simulink model "FUZZY_T2_ADRC_P3DX"  (R2024b)
settings: Solver=FixedStepAuto  StartTime=0.0  StopTime=16  FixedStep=0.01  RelTol=1e-2
libraries: fuzblock x2, simulink x1
settings Model: Creator=Dell  LastModifiedBy=Dell
settings DebuggingCC: AlgebraicLoopMsg=none  SigSpecEnsureSampleTimeMsg=none
settings RTWCC: GPUComputeCapability=3.5

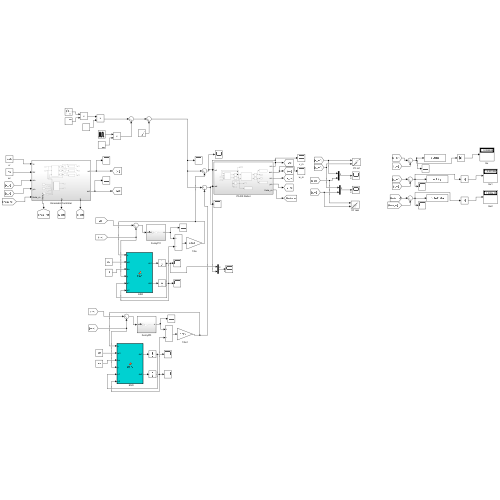
[thumbnail: Simulink's stored preview of the top-level diagram]
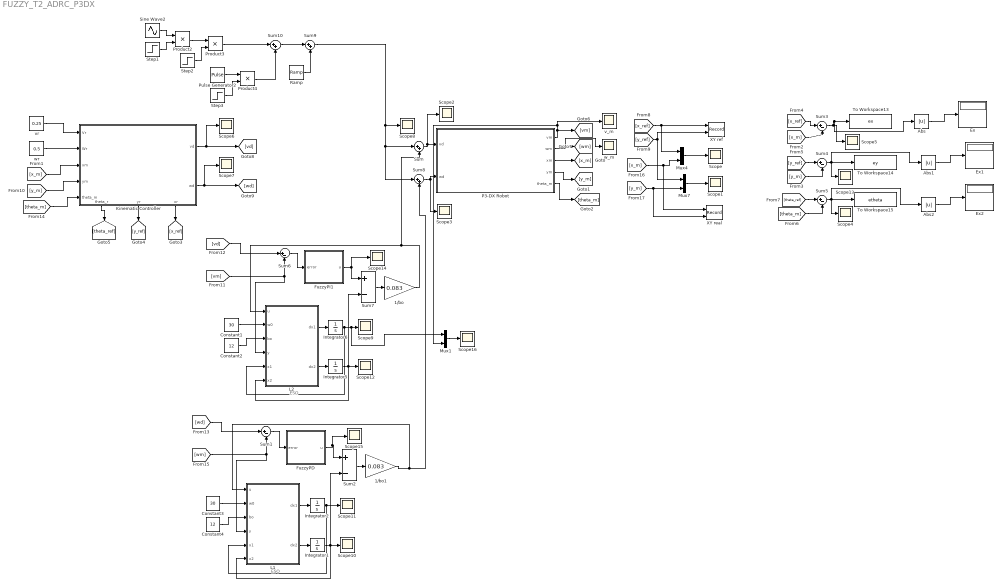
== system FUZZY_T2_ADRC_P3DX ==
  note: ESO
  note: ESO
  1/bo : Gain  Gain=0.083
  1/bo1 : Gain  Gain=0.083
  Abs : Abs  SaturateOnIntegerOverflow=off
  Abs1 : Abs  SaturateOnIntegerOverflow=off
  Abs2 : Abs  SaturateOnIntegerOverflow=off
  Constant1 : Constant  Value=30
  Constant2 : Constant  Value=12
  Constant3 : Constant  Value=30
  Constant4 : Constant  Value=12
  Ex : Display
  Ex1 : Display
  Ex2 : Display
  FuzzyPD : Subsystem
  FuzzyPI1 : Subsystem
  Integrator{1..2,5..6} (4 alike) : Integrator
  Kinematic Controller : Subsystem
      settings: PortSchema="{\"entries\":[{\"content\":{\"sides\":[{\"content\":{\"connectorIds\":[\"In1\",\"In2\",\"In3\",\"In4\",\"In5\"]},\"type\":\"ConnectorPlacement.EquallySpacedRectSide\",\"uuid\":\"1dde3c4d-b362-4c98-bff5-173134d67a18\"},{\"content\":{\"connectorIds\":[\"Out1\",\"Out2\"],\"side\":\"RIGHT\"},\"type\":\"ConnectorPlacement.EquallySpacedRectSide\",\"uuid\":\"28a7b07a-1542-4ec6-930a-70e18e33702f\"},{\"content\":{\"side\":\"TOP\"},\"type\":\"ConnectorPlacement.EquallySpacedRectSide\",\"uuid\":\"fddfb50e-6b1f-4e7e-bd72-f809cd3d8285\"},{\"content\":{\"connectorIds\":[\"Out3\",\"Out4\",\"Out5\"],\"side\":\"BOTTOM\"},\"type\":\"ConnectorPlacement.EquallySpacedRectSide\",\"uuid\":\"0cbc9f95-9386-4a92-999a-6cc6855b0431\"}]},\"type\":\"ConnectorPlacement.EquallySpacedConnector\",\"uuid\":\"21383b85-61ab-4832-be46-2fedf08e757e\"}],\"packageUris\":[\"http://schema.mathworks.com/mf0/Connector/R2020b\"],\"version\":\"1.0\"}"
  L1 : MATLAB Function  TreatAsAtomicUnit=on
  L2 : MATLAB Function  TreatAsAtomicUnit=on
  Mux1 : Mux  Inputs=2
  Mux4 : Mux  Inputs=2
  Mux7 : Mux  Inputs=2
  P3-DX Robot : Subsystem
  Product2 : Product
  Product3 : Product
  Product4 : Product
  Pulse Generator2 : DiscretePulseGenerator  PulseType=Time based  Amplitude=4  Period=1  PulseWidth=35  PhaseDelay=9.7
  Ramp : simulink/Sources/Ramp  slope=1  start=14.3  InitialOutput=0
  Scope{,1..16} (17 alike) : Scope
  Sine Wave2 : Sin  Amplitude=4  Frequency=2  SampleTime=0
  Step1 : Step  Time=3.2  SampleTime=0
  Step2 : Step  Time=9.4  Before=1  After=0  SampleTime=0
  Step3 : Step  Time=14  Before=1  After=0  SampleTime=0
  Sum{,8..10} (4 alike) : Sum  Inputs=|++
  Sum{1,3..6} (5 alike) : Sum  Inputs=|+-
  Sum2 : Sum  Inputs=+-
  Sum7 : Sum  Inputs=+-
  To Workspace13 : ToWorkspace  VariableName=ex  SaveFormat=Timeseries  SampleTime=-1
  To Workspace14 : ToWorkspace  VariableName=ey  SaveFormat=Timeseries  SampleTime=-1
  To Workspace15 : ToWorkspace  VariableName=etheta  SaveFormat=Timeseries  SampleTime=-1
  XY real : Record  FileSettingsInternal="{\"entries\":[{\"content\":{\"excelSettings\":{\"content\":{},\"type\":\"Streamout.ExcelSettings\"}},\"type\":\"Streamout.FileSettingStorage\",\"uuid\":\"\"}],\"packageUris\":[\"http:\\/\\/schema.mathworks.com\\/mf0\\/streamout_blocks\\/R2020a\"],\"version\":\"1.0\"}"  Layout=[1 1]  SignalsInternal="{\"entries\":[{\"content\":{\"signals\":[{\"content\":{\"blockPath\":[],\"dimensions\":[1],\"domain\":\"\",\"lineColor\":\"#139fff\",\"lineWidth\":2,\"port\":1,\"sid\":[\"\"],\"signalID\":1,\"signalName\":\"From16\"},\"type\":\"RecordBlkView.Signal\",\"uuid\":\"\"},{\"content\":{\"blockPath\":[],\"dimensions\":[1],\"domain\":\"\",\"lineColor\":\"#ff6929\",\"lineWidth\":2,\"port\":2,\"sid\":[\"\"],\"signalID\":2,\"signalName\":\"From17\"},\"type\":\"RecordBlkView.Signal\",\"uuid\":\"\"}]},\"type\":\"RecordBlkView.InputSignals\",\"uuid\":\"\"}],\"packageUris\":[\"http:\\/\\/schema.mathworks.com\\/mf0\\/streamout_blocks\\/R2020a\"],\"version\":\"1.0\"}"  VisualizationBindings="{\"xyplotplugin\":{\"info\":[{\"series\":[],\"subplotID\":1}]}}"  CompatibilityTag=XY
  XY ref : Record  FileSettingsInternal="{\"entries\":[{\"content\":{\"excelSettings\":{\"content\":{},\"type\":\"Streamout.ExcelSettings\"}},\"type\":\"Streamout.FileSettingStorage\",\"uuid\":\"\"}],\"packageUris\":[\"http:\\/\\/schema.mathworks.com\\/mf0\\/streamout_blocks\\/R2020a\"],\"version\":\"1.0\"}"  Layout=[1 1]  SignalsInternal="{\"entries\":[{\"content\":{\"signals\":[{\"content\":{\"blockPath\":[],\"dimensions\":[1],\"domain\":\"\",\"lineColor\":\"#b746ff\",\"lineWidth\":2,\"port\":1,\"sid\":[\"\"],\"signalID\":1,\"signalName\":\"From8\"},\"type\":\"RecordBlkView.Signal\",\"uuid\":\"\"},{\"content\":{\"blockPath\":[],\"dimensions\":[1],\"domain\":\"\",\"lineColor\":\"#64d413\",\"lineWidth\":2,\"port\":2,\"sid\":[\"\"],\"signalID\":2,\"signalName\":\"From9\"},\"type\":\"RecordBlkView.Signal\",\"uuid\":\"\"}]},\"type\":\"RecordBlkView.InputSignals\",\"uuid\":\"\"}],\"packageUris\":[\"http:\\/\\/schema.mathworks.com\\/mf0\\/streamout_blocks\\/R2020a\"],\"version\":\"1.0\"}"  VisualizationBindings="{\"xyplotplugin\":{\"info\":[{\"series\":[],\"subplotID\":1}]}}"  CompatibilityTag=XY
  v_m : Scope
  vr : Constant  Value=0.25
  w_m : Scope
  wr : Constant  Value=0.5
  wires:
  Abs1/1 -> Ex1/1
  Abs/1 -> Ex/1
  [y_ref] -> Sum4/1
  [x_m] -> Sum3/2
  [theta_m] -> Sum5/2
  Sum5/1 -> Abs2/1, Scope4/1, To Workspace15/1
  Sum3/1 -> Abs/1, To Workspace13/1, Scope5/1
  [theta_ref] -> Sum5/1
  Abs2/1 -> Ex2/1
  [y_m] -> Sum4/2
  [x_ref] -> Sum3/1
  Sum4/1 -> Abs1/1, Scope13/1, To Workspace14/1
  Mux4/1 -> Scope/1
  Mux7/1 -> Scope1/1
  [y_ref] -> XY ref/2, Mux7/1
  [x_ref] -> XY ref/1, Mux4/1
  [x_m] -> XY real/1, Mux4/2
  [y_m] -> XY real/2, Mux7/2
  [y_m] -> Kinematic Controller/4(ym)
  vr/1 -> Kinematic Controller/1(Vr)
  wr/1 -> Kinematic Controller/2(Wr)
  [x_m] -> Kinematic Controller/3(xm)
  [theta_m] -> Kinematic Controller/5(theta_m)
  P3-DX Robot/3(xm) -> [x_m]
  P3-DX Robot/4(ym) -> [y_m]
  P3-DX Robot/5(theta_m) -> [theta_m]
  Kinematic Controller/5(xr) -> [x_ref]
  Kinematic Controller/4(yr) -> [y_ref]
  Kinematic Controller/3(theta_r) -> [theta_ref]
  P3-DX Robot/1(vm) -> Mux1/2, v_m/1, [vm]
  Kinematic Controller/2(wd) -> [wd], Scope7/1
  P3-DX Robot/2(wm) -> w_m/1, [wm]
  Kinematic Controller/1(vd) -> [vd], Scope6/1
  1/bo/1 -> Sum/2, L2/1(u)
  Constant2/1 -> L2/3(bo)
  [vd] -> Sum6/1
  Integrator6/1 -> L2/5(x1), Mux1/1, Scope9/1
  Sum7/1 -> 1/bo/1
  [vm] -> L2/4(y), Sum6/2
  Constant1/1 -> L2/2(w0)
  Integrator5/1 -> Sum7/2, Scope12/1, L2/6(x2)
  L2/2(dx2) -> Integrator5/1
  L2/1(dx1) -> Integrator6/1
  L1/2(dx2) -> Integrator1/1
  Integrator1/1 -> Sum2/2, Scope10/1, L1/6(x2)
  [wm] -> L1/4(y), Sum1/2
  Constant3/1 -> L1/2(w0)
  Sum2/1 -> 1/bo1/1
  Integrator2/1 -> L1/5(x1), Scope11/1
  L1/1(dx1) -> Integrator2/1
  [wd] -> Sum1/1
  Constant4/1 -> L1/3(bo)
  1/bo1/1 -> Sum8/2, L1/1(u)
  Sum/1 -> Scope2/1, P3-DX Robot/1(vd)
  Sum8/1 -> Scope3/1, P3-DX Robot/2(wd)
  Sum1/1 -> FuzzyPD/1(error)
  FuzzyPD/1(u) -> Scope15/1, Sum2/1
  Sum9/1 -> Sum8/1, Sum/1, Scope8/1
  Pulse Generator2/1 -> Product4/1
  Ramp/1 -> Sum9/2
  Sine Wave2/1 -> Product2/1
  Step1/1 -> Product2/2
  Step2/1 -> Product3/2
  Product4/1 -> Sum10/2
  Sum10/1 -> Sum9/1
  Step3/1 -> Product4/2
  Product3/1 -> Sum10/1
  Product2/1 -> Product3/1
  Sum6/1 -> FuzzyPI1/1(error)
  FuzzyPI1/1(u) -> Sum7/1, Scope14/1
  Mux1/1 -> Scope16/1

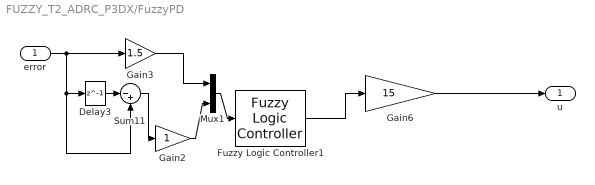
== system FUZZY_T2_ADRC_P3DX/FuzzyPD ==
  error : Inport
  Delay3 : Delay  DelayLength=1  InitialCondition=0
  Fuzzy Logic Controller1 : fuzblock/Fuzzy Logic  Controller  FIS='PI_type2.fis'  OutputSampleNumber=101  DataType=double  FuzzifiedInputs=off  RuleFiringStrengths=off  RuleOutputs=off  AggregatedOutputs=off  SimulateUsing=Interpreted execution  OutOfRangeInputValueMessage=warning  NoRuleFiredMessage=warning  EmptyOutputFuzzySetMessage=warning
  Gain2 : Gain
  Gain3 : Gain  Gain=1.5
  Gain6 : Gain  Gain=15
  Mux1 : Mux  Inputs=2
  Sum11 : Sum  Inputs=|-+
  u : Outport
  wires:
  error/1 -> Gain3/1, Sum11/2, Delay3/1
  Delay3/1 -> Sum11/1
  Sum11/1 -> Gain2/1
  Gain2/1 -> Mux1/2
  Mux1/1 -> Fuzzy Logic Controller1/1
  Fuzzy Logic Controller1/1 -> Gain6/1
  Gain3/1 -> Mux1/1
  Gain6/1 -> u/1

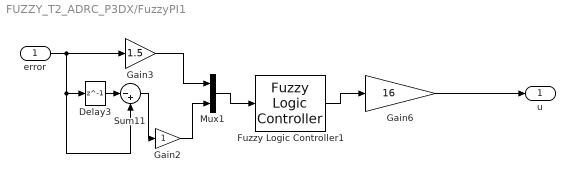
== system FUZZY_T2_ADRC_P3DX/FuzzyPI1 ==
  error : Inport
  Delay3 : Delay  DelayLength=1  InitialCondition=0
  Fuzzy Logic Controller1 : fuzblock/Fuzzy Logic  Controller  FIS='PI_type2.fis'  OutputSampleNumber=101  DataType=double  FuzzifiedInputs=off  RuleFiringStrengths=off  RuleOutputs=off  AggregatedOutputs=off  SimulateUsing=Interpreted execution  OutOfRangeInputValueMessage=warning  NoRuleFiredMessage=warning  EmptyOutputFuzzySetMessage=warning
  Gain2 : Gain
  Gain3 : Gain  Gain=1.5
  Gain6 : Gain  Gain=16
  Mux1 : Mux  Inputs=2
  Sum11 : Sum  Inputs=|-+
  u : Outport
  wires:
  error/1 -> Gain3/1, Sum11/2, Delay3/1
  Delay3/1 -> Sum11/1
  Sum11/1 -> Gain2/1
  Gain2/1 -> Mux1/2
  Mux1/1 -> Fuzzy Logic Controller1/1
  Fuzzy Logic Controller1/1 -> Gain6/1
  Gain3/1 -> Mux1/1
  Gain6/1 -> u/1

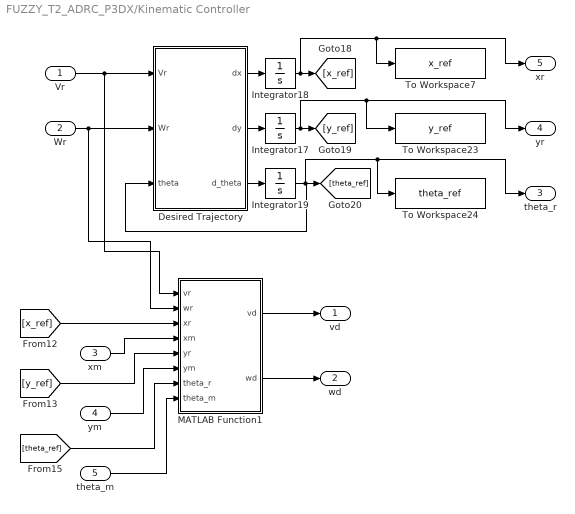
== system FUZZY_T2_ADRC_P3DX/Kinematic Controller ==
  Vr : Inport
  Wr : Inport  Port=2
  xm : Inport  Port=3
  ym : Inport  Port=4
  theta_m : Inport  Port=5
  " Desired Trajectory" : MATLAB Function  TreatAsAtomicUnit=on
  Integrator17 : Integrator  InitialCondition=-0.5
  Integrator18 : Integrator
  Integrator19 : Integrator
  MATLAB Function1 : MATLAB Function  TreatAsAtomicUnit=on
  To Workspace23 : ToWorkspace  VariableName=y_ref  SaveFormat=Timeseries  SampleTime=-1
  To Workspace24 : ToWorkspace  VariableName=theta_ref  SaveFormat=Timeseries  SampleTime=-1
  To Workspace7 : ToWorkspace  VariableName=x_ref  SaveFormat=Timeseries  SampleTime=-1
  vd : Outport
  wd : Outport  Port=2
  theta_r : Outport  Port=3
  yr : Outport  Port=4
  xr : Outport  Port=5
  wires:
  " Desired Trajectory"/3(d_theta) -> Integrator19/1
  Integrator19/1 -> theta_r/1, To Workspace24/1, " Desired Trajectory"/3(theta), [theta_ref]
  Integrator18/1 -> xr/1, To Workspace7/1, [x_ref]
  Vr/1 -> MATLAB Function1/1(vr), " Desired Trajectory"/1(Vr)
  " Desired Trajectory"/1(dx) -> Integrator18/1
  Wr/1 -> MATLAB Function1/2(wr), " Desired Trajectory"/2(Wr)
  MATLAB Function1/1(vd) -> vd/1
  MATLAB Function1/2(wd) -> wd/1
  " Desired Trajectory"/2(dy) -> Integrator17/1
  Integrator17/1 -> yr/1, To Workspace23/1, [y_ref]
  [x_ref] -> MATLAB Function1/3(xr)
  xm/1 -> MATLAB Function1/4(xm)
  [y_ref] -> MATLAB Function1/5(yr)
  ym/1 -> MATLAB Function1/6(ym)
  [theta_ref] -> MATLAB Function1/7(theta_r)
  theta_m/1 -> MATLAB Function1/8(theta_m)

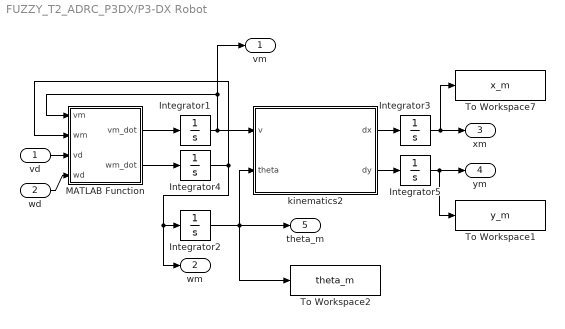
== system FUZZY_T2_ADRC_P3DX/P3-DX Robot ==
  vd : Inport
  wd : Inport  Port=2
  Integrator{1..5} (5 alike) : Integrator
  MATLAB Function : MATLAB Function  TreatAsAtomicUnit=on
  To Workspace1 : ToWorkspace  VariableName=y_m  SaveFormat=Timeseries  SampleTime=-1
  To Workspace2 : ToWorkspace  VariableName=theta_m  SaveFormat=Timeseries  SampleTime=-1
  To Workspace7 : ToWorkspace  VariableName=x_m  SaveFormat=Timeseries  SampleTime=-1
  kinematics2 : MATLAB Function  TreatAsAtomicUnit=on
  vm : Outport
  wm : Outport  Port=2
  xm : Outport  Port=3
  ym : Outport  Port=4
  theta_m : Outport  Port=5
  wires:
  Integrator2/1 -> To Workspace2/1, theta_m/1, kinematics2/2(theta)
  MATLAB Function/1(vm_dot) -> Integrator1/1
  MATLAB Function/2(wm_dot) -> Integrator4/1
  Integrator1/1 -> kinematics2/1(v), MATLAB Function/1(vm), vm/1
  Integrator3/1 -> To Workspace7/1, xm/1
  Integrator4/1 -> MATLAB Function/2(wm), Integrator2/1, wm/1
  kinematics2/2(dy) -> Integrator5/1
  vd/1 -> MATLAB Function/3(vd)
  kinematics2/1(dx) -> Integrator3/1
  wd/1 -> MATLAB Function/4(wd)
  Integrator5/1 -> To Workspace1/1, ym/1

== matlab function FUZZY_T2_ADRC_P3DX/Kinematic Controller/MATLAB Function1 ==
  data: vr input; wr input; xr input; vd output; xm input; yr input; ym input; theta_r input; theta_m input; wd output
function [vd, wd] = fcn(vr, wr, xr, xm, yr, ym, theta_r, theta_m)
ex = ((xr - xm) * cos(theta_m)) + ((yr - ym) * sin(theta_m));
ey = - ((xr - xm) * sin(theta_m)) + ((yr - ym) * cos(theta_m));

etheta = theta_r - theta_m;

kx = 0.8;
ky = 0.8;
kth = 0.8;

vd = (kx * ex) + (vr * cos(etheta));
wd = (ky * vr * ey ) + wr + (kth * sin(etheta));

== matlab function FUZZY_T2_ADRC_P3DX/P3-DX Robot/MATLAB Function ==
  data: vm input; vm_dot output; wm input; wm_dot output; vd input; wd input
function[vm_dot, wm_dot] = fcn(vm,wm,vd,wd)
k1 = 0.24089;
k2 = 0.2424;
k3 = -0.00093603;
k4 = 0.99629;
k5 = -0.0057256;
k6 = 1;


vm_dot = ((k3/k1) * (wm*wm)) - ((k4/k1) * vm) + (vd/k1);
wm_dot = - ((k5/k2) * (vm*wm)) - ((k6/k2) * wm) + (wd/k2);

== matlab function FUZZY_T2_ADRC_P3DX/P3-DX Robot/kinematics2 ==
  data: v input; dx output; dy output; theta input
function [dx, dy] = kinematics(v, theta)


dx =  v .* cos(theta);
dy =  v .* sin(theta);

== matlab function FUZZY_T2_ADRC_P3DX/L1 ==
  data: dx1 output; dx2 output; u input; w0 input; bo input; y input; x1 input; x2 input
function [dx1,dx2] =ESO(u,w0,bo,y, x1,x2)

%bo=[15.5311 -3.5587;
   % -3.5587 15.5311];
% l1, l2, l3 ARE THE OBSERVER GAINS IN ESO calcualated using w0
L1=2*w0;   
L2=w0^2;

e = x1-y;

dx1 = x2 + (bo * u) - (L1 * e);
dx2 = - (L2 * e);

%dx1 = reshape(dx1, 1, []);
%dx2 = reshape(dx2, 1, []);

== matlab function FUZZY_T2_ADRC_P3DX/L2 ==
  data: dx1 output; dx2 output; u input; w0 input; bo input; y input; x1 input; x2 input
function [dx1,dx2] =ESO(u,w0,bo,y, x1,x2)

%bo=[15.5311 -3.5587;
   % -3.5587 15.5311];
% l1, l2, l3 ARE THE OBSERVER GAINS IN ESO calcualated using w0
L1=2*w0;   
L2=w0^2;

e = x1-y;

dx1 = x2 + (bo * u) - (L1 * e);
dx2 = - (L2 * e);

%dx1 = reshape(dx1, 1, []);
%dx2 = reshape(dx2, 1, []);

== matlab function FUZZY_T2_ADRC_P3DX/Kinematic Controller/ Desired Trajectory ==
  data: Vr input; Wr input; theta input; dx output; dy output; d_theta output
function [dx, dy, d_theta] = desiredtraj(Vr, Wr, theta)
    dx = cos(theta) * Vr ;
    dy = sin(theta) * Vr ;
    d_theta = Wr;
    

end
